simulink model "INPUT"  (R2024b)
settings: Solver=FixedStepDiscrete  StartTime=0.0  StopTime=1  FixedStep=0.001  RelTol=1e-3  EnableMultiTasking=on
settings Model: DataDictionary=Master_Dictionary.sldd  EnableAccessToBaseWorkspace=off  Creator=torni  LastModifiedBy=oxbro
settings SolverCC: AlgebraicLoopSolver=TrustRegion
settings DataIOCC: ReturnWorkspaceOutputs=off
settings OptimizationCC: DefaultParameterBehavior=Inlined  EnhancedBackFolding=on  PassReuseOutputArgsAs=Individual arguments  ZeroExternalMemoryAtStartup=off  ZeroInternalMemoryAtStartup=off  MaxStackSize=512  OptimizeBlockOrder=speed  DifferentSizesBufferReuse=on  OptimizationCustomize=off  EfficientTunableParamExpr=on
settings DebuggingCC: ParameterTunabilityLossMsg=error  UnconnectedInputMsg=warning  UnconnectedOutputMsg=warning  UnconnectedLineMsg=warning  ArithmeticOperatorsInVariantConditions=warning
settings HardwareCC: ProdBitPerPointer=32  ProdBitPerSizeT=32  ProdBitPerPtrDiffT=32  ProdLargestAtomicInteger=Long  ProdLargestAtomicFloat=Double  ProdWordSize=32  ProdLongLongMode=on  ProdHWDeviceType=ARM Compatible->ARM Cortex-M
settings ModelReferenceCC: EnableRefExpFcnMdlSchedulingChecks=on
settings SFSimCC: MATLABDynamicMemAlloc=off  CustomCodeUndefinedFunction=UseInterfaceOnly
settings RTWCC: Description=Embedded Coder  SystemTargetFile=ert.tlc  HardwareBoard=STM32H7xx Based (Single-core)  TemplateMakefile=ert_default_tmf  CustomHeaderCode="#include \"stm32h7xx_ll_tim.h\""  CustomInitializer=LL_TIM_EnableCounter(TIM2);  Toolchain=GNU Tools for ARM Embedded Processors  GPUComputeCapability=3.5
settings CodeAppCC: ForceParamTrailComments=on  IgnoreCustomStorageClasses=off  OperatorAnnotations=on  SimulinkDataObjDesc=on  SFDataObjDesc=on  InsertBlockDesc=on
settings ERTTargetCC: TargetLangStandard=C99 (ISO)  CodeReplacementLibrary=ARM Cortex-M  ExtModeTransport=3  ExtModeStaticAlloc=on  ExtModeStaticAllocSize=2048  ExtModeMexFile=ext_xcp  ExtModeIntrfLevel=Level2 - Open

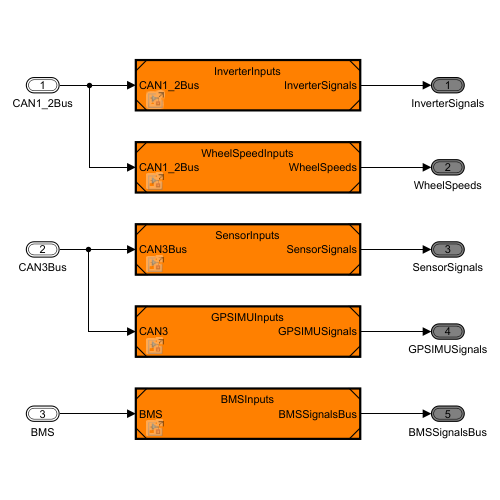
[thumbnail: Simulink's stored preview of the top-level diagram]
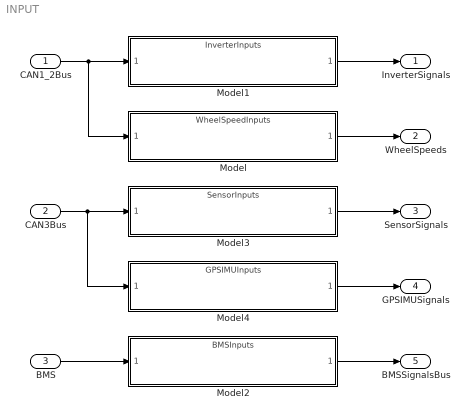
== system INPUT ==
  CAN1_2Bus : Inport  OutDataTypeStr=Bus: CAN1_2Bus
  CAN3Bus : Inport  Port=2  OutDataTypeStr=Bus: CAN3Bus
  BMS : Inport  Port=3  OutDataTypeStr=Bus: BMS
  Model : ModelReference  ModelNameDialog=WheelSpeedInputs.slx  SimulationMode=Normal  ModelReferenceVersion=13.0
  Model1 : ModelReference  ModelNameDialog=InverterInputs.slx  SimulationMode=Normal  ModelReferenceVersion=13.0
  Model2 : ModelReference  ModelNameDialog=BMSInputs.slx  SimulationMode=Normal  ModelReferenceVersion=13.0
  Model3 : ModelReference  ModelNameDialog=SensorInputs.slx  SimulationMode=Normal  ModelReferenceVersion=13.0
  Model4 : ModelReference  ModelNameDialog=GPSIMUInputs.slx  SimulationMode=Normal  ModelReferenceVersion=13.0
  InverterSignals : Outport  OutDataTypeStr=Bus: InverterSignals  VectorParamsAs1DForOutWhenUnconnected=off
  WheelSpeeds : Outport  Port=2  OutDataTypeStr=Bus: WheelSpeeds  VectorParamsAs1DForOutWhenUnconnected=off
  SensorSignals : Outport  Port=3  OutDataTypeStr=Bus: SensorSignals  VectorParamsAs1DForOutWhenUnconnected=off
  GPSIMUSignals : Outport  Port=4  OutDataTypeStr=Bus: GPSIMUSignals  VectorParamsAs1DForOutWhenUnconnected=off
  BMSSignalsBus : Outport  Port=5  OutDataTypeStr=Bus: BMSSignals  VectorParamsAs1DForOutWhenUnconnected=off
  wires:
  Model/1 -> WheelSpeeds/1
  Model1/1 -> InverterSignals/1
  CAN3Bus/1 -> Model4/1, Model3/1
  CAN1_2Bus/1 -> Model1/1, Model/1
  Model2/1 -> BMSSignalsBus/1
  BMS/1 -> Model2/1
  Model3/1 -> SensorSignals/1
  Model4/1 -> GPSIMUSignals/1
